simulink model "controller_angular_rates"  (R2020a)
settings: Solver=FixedStepAuto  StartTime=0.0  StopTime=10.0  FixedStep=1/sim_freq  RelTol=1e-3
undefined symbols (not defined in the file): hover_perc
settings Model: Creator=francois  LastModifiedBy=murray
settings DebuggingCC: ModelReferenceExtraNoncontSigs=none

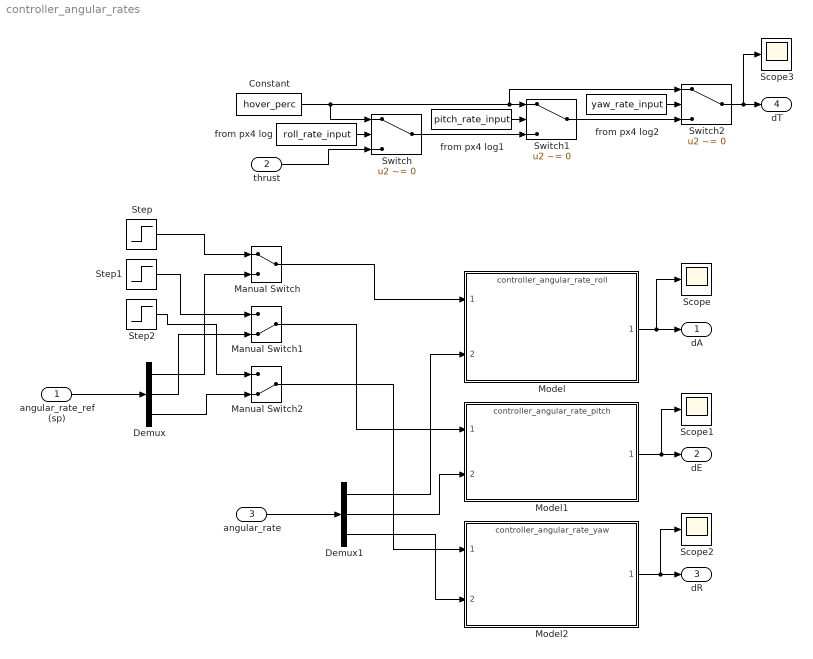
== system controller_angular_rates ==
  angular_rate_ref (sp) : Inport
  thrust : Inport  Port=2
  "angular_rate " : Inport  Port=3
  " from px4 log1" : FromWorkspace  VariableName=pitch_rate_input
  Constant : Constant  Value=hover_perc
  Demux : Demux  Outputs=3
  Demux1 : Demux  Outputs=3
  Manual Switch : ManualSwitch
  Manual Switch1 : ManualSwitch  CurrentSetting=0
  Manual Switch2 : ManualSwitch  CurrentSetting=0
  Model : ModelReference  ModelNameDialog=controller_angular_rate_roll.slx  SimulationMode=Normal  ModelReferenceVersion=1.14
  Model1 : ModelReference  ModelNameDialog=controller_angular_rate_pitch.slx  SimulationMode=Normal  ModelReferenceVersion=1.14
  Model2 : ModelReference  ModelNameDialog=controller_angular_rate_yaw.slx  SimulationMode=Normal  ModelReferenceVersion=1.15
  Scope{,1..3} (4 alike) : Scope
  Step : Step  Time=0.5  After=0  SampleTime=0
  Step1 : Step  Time=0.5  After=0.09  SampleTime=0
  Step2 : Step  Time=0.5  After=0  SampleTime=0
  Switch : Switch  Criteria=u2 ~= 0
  Switch1 : Switch  Criteria=u2 ~= 0
  Switch2 : Switch  Criteria=u2 ~= 0
  from px4 log : FromWorkspace  VariableName=roll_rate_input
  from px4 log2 : FromWorkspace  VariableName=yaw_rate_input
  dA : Outport
  dE : Outport  Port=2
  dR : Outport  Port=3
  dT : Outport  Port=4  VectorParamsAs1DForOutWhenUnconnected=off
  wires:
  angular_rate_ref (sp)/1 -> Demux/1
  "angular_rate "/1 -> Demux1/1
  Demux1/1 -> Model/2
  Demux1/2 -> Model1/2
  Demux1/3 -> Model2/2
  Model/1 -> Scope/1, dA/1
  Model1/1 -> Scope1/1, dE/1
  Model2/1 -> Scope2/1, dR/1
  Switch1/1 -> Switch2/3
  Switch2/1 -> dT/1, Scope3/1
  thrust/1 -> Switch/3
  from px4 log/1 -> Switch/2
  Constant/1 -> Switch/1, Switch2/1, Switch1/1
  Switch/1 -> Switch1/3
  from px4 log2/1 -> Switch2/2
  " from px4 log1"/1 -> Switch1/2
  Step/1 -> Manual Switch/1
  Demux/1 -> Manual Switch/2
  Demux/2 -> Manual Switch1/2
  Step1/1 -> Manual Switch1/1
  Demux/3 -> Manual Switch2/2
  Step2/1 -> Manual Switch2/1
  Manual Switch/1 -> Model/1
  Manual Switch1/1 -> Model1/1
  Manual Switch2/1 -> Model2/1
